simulink library "lib_GenTools_PolynomialFit"  (R2015a)
settings: Solver=ode45  StartTime=0.0  StopTime=10.0  RelTol=1e-3
settings Model: Creator=jlkratz  LastModifiedBy=jlkratz

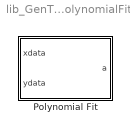
== system lib_GenTools_PolynomialFit ==
  Polynomial Fit : Subsystem  mask(TSAT: Polynomial Fit){N_M=5, BN_M=double(gcb)}
      mask prompts: N_M "N_M - Power of the polynomial (must be a positive integer that is less than or equal to the number of data points )"; BN_M "BN_M - Block Name"
      mask help:
      | This block allow for on-the-fly polynomial fits to data. The power of the polynomial is given as a parameter and the data is the inputs. The output is the polynomial coefficients:
      |
      | y(x) = a0+ a1*x + a2*x^2 + ... + aN*x^N
      |
      | a = [a0 a1 a2 ... aN]
      |
      | See the help menu for more details.
      mask init:
      | if N_M < 1 || rem(N_M,1) > 0
      |     N_M = max([round(N_M) 1]);
      |     fprintf('Error in %s: N_M must be an integer greater than or equal to 1. N_M has been rounded to the closest integer or set to 1, whichever is closer to the input value while still satisfying the requirements.\n',char(BN_M)); 
      | end
      mask Help: web(which('GenTools_TSAT_PolynomialFit.html'),'-helpbrowser')

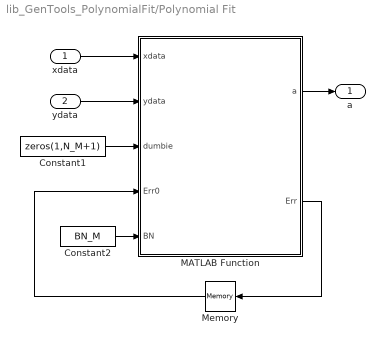
== system lib_GenTools_PolynomialFit/Polynomial Fit ==
  xdata : Inport
  ydata : Inport  Port=2
  Constant1 : Constant  Value=zeros(1,N_M+1)
  Constant2 : Constant  Value=BN_M
  MATLAB Function : MATLAB Function  TreatAsAtomicUnit=on
  Memory : Memory  X0=zeros(1,11)
  a : Outport
  wires:
  Constant2/1 -> MATLAB Function/5(BN)
  Memory/1 -> MATLAB Function/4(Err0)
  MATLAB Function/2(Err) -> Memory/1
  Constant1/1 -> MATLAB Function/3(dumbie)
  ydata/1 -> MATLAB Function/2(ydata)
  xdata/1 -> MATLAB Function/1(xdata)
  MATLAB Function/1(a) -> a/1

== matlab function lib_GenTools_PolynomialFit/Polynomial Fit/MATLAB Function ==
  data: xdata input; a output; ydata input; dumbie input; Err0 input; Err output; BN input
function [a,Err] = PolynomialFit(xdata,ydata,dumbie,Err0,BN)
%#codegen

%Power of the polynomial
N = length(dumbie)-1;

%Error/Warning Checking 
Err = Err0;
ErrNum = 1;
%xdata is a 1-D Array
if min(size(xdata)) ~= 1 && Err(ErrNum) == 0
    fprintf('Warning in %s: xdata must be a 1-D array\n',char(BN));
    Err(ErrNum) = 1;
end
ErrNum = ErrNum + 1;
%ydata is a 1-D Array
if min(size(ydata)) ~= 1 && Err(ErrNum) == 0
    fprintf('Warning in %s: ydata must be a 1-D array\n',char(BN));
    Err(ErrNum) = 1;
end
ErrNum = ErrNum + 1;
%xdata and ydata are the same length 
if length(xdata) ~= length(ydata) && Err(ErrNum) == 0
    fprintf('Warning in %s: xdata and ydata must be the same length\n',char(BN));
    Err(ErrNum) = 1;
end
ErrNum = ErrNum + 1;
%Power of polynomial is less than
if N > length(xdata) && Err(ErrNum) == 0
    fprintf('Warning in %s: N_M must be less than or equal to the number of data points in xdata\n',char(BN));
    Err(ErrNum) = 1;
end
ErrNum = ErrNum + 1;
%xdata has all real elements
if min(isreal(xdata)) < 1 && Err(ErrNum) == 0
    fprintf('Warning in %s: xdata must have all real elements\n',char(BN));
    Err(ErrNum) = 1;
end
ErrNum = ErrNum + 1;
%ydata has all real elements
if min(isreal(ydata)) < 1 && Err(ErrNum) == 0
    fprintf('Warning in %s: ydata must have all real elements\n',char(BN));
    Err(ErrNum) = 1;
end
ErrNum = ErrNum + 1;
%xdata has all finite elements
if max(isinf(xdata)) == 1 && Err(ErrNum) == 0
    fprintf('Warning in %s: xdata must have all finite elements\n',char(BN));
    Err(ErrNum) = 1;
end
ErrNum = ErrNum + 1;
%ydata has all finite elements
if max(isinf(ydata)) == 1 && Err(ErrNum) == 0
    fprintf('Warning in %s: ydata must have all finite elements\n',char(BN));
    Err(ErrNum) = 1;
end
ErrNum = ErrNum + 1;
%xdata has all non-NaN elements
if max(isnan(xdata)) == 1 && Err(ErrNum) == 0
    fprintf('Warning in %s: xdata must have all non-NaN elements\n',char(BN));
    Err(ErrNum) = 1;
end
ErrNum = ErrNum + 1;
%ydata has all non-NaN elements
if max(isnan(ydata)) == 1 && Err(ErrNum) == 0
    fprintf('Warning in %s: ydata must have all non-NaN elements\n',char(BN));
    Err(ErrNum) = 1;
end
ErrNum = ErrNum + 1;
%xdata is monotonically increasing
diffxdata = diff(xdata);
if min(diffxdata) <= 0 && Err(ErrNum) == 0
    fprintf('Warning in %s: xdata must be monotonically increasing\n',char(BN));
    Err(ErrNum) = 1;
end

%Calculations
a = zeros(1,N+1);
A = polyfit(xdata,ydata,N);
A = fliplr(A);
for i = 1:N+1
    a(i) = A(i);
end
